simulink model "Motor_control"  (R2025b)
settings: Solver=ode45  StartTime=0.0  StopTime=3  MaxStep=1e-5  RelTol=1e-5
undefined symbols (not defined in the file): C, F, fc, G, K, K_I, L, T, x_r
settings Model: Creator=noeliarosales  LastModifiedBy=noeliarosales

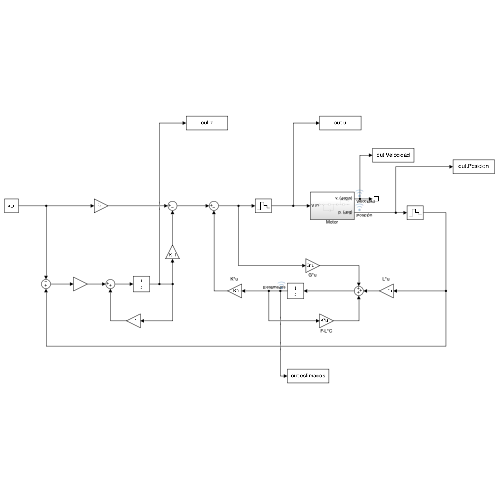
[thumbnail: Simulink's stored preview of the top-level diagram]
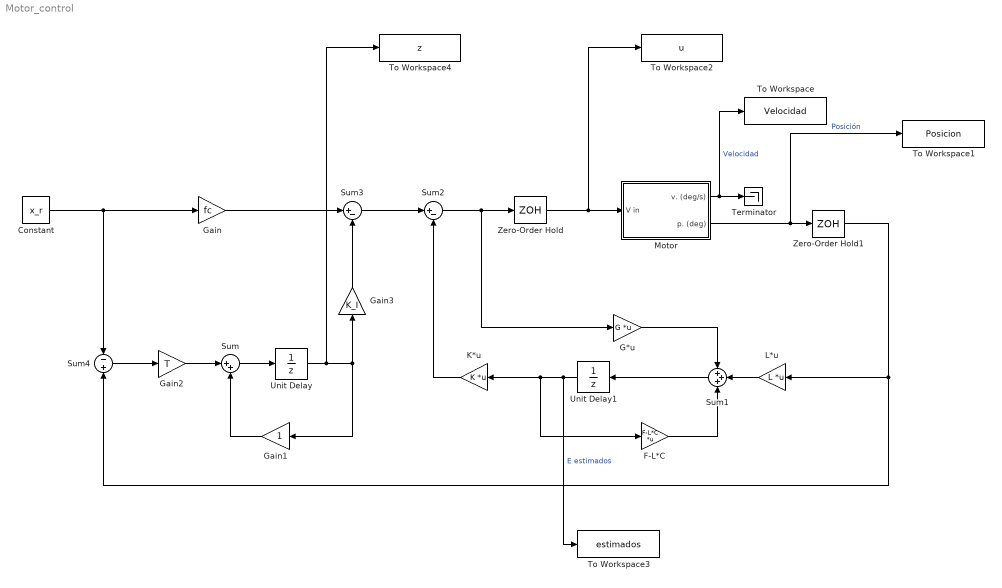
== system Motor_control ==
  Constant : Constant  Value=x_r
  F-L*C : Gain  Gain=F-L*C  Multiplication=Matrix(K*u)
  G*u : Gain  Gain=G  Multiplication=Matrix(K*u)
  Gain : Gain  Gain=fc
  Gain1 : Gain
  Gain2 : Gain  Gain=T
  Gain3 : Gain  Gain=K_I
  K*u : Gain  Gain=K  Multiplication=Matrix(K*u)
  L*u : Gain  Gain=L  Multiplication=Matrix(K*u)
  Motor : Subsystem
  Sum : Sum  Inputs=|++
  Sum1 : Sum  Inputs=+++
  Sum2 : Sum  Inputs=|+-
  Sum3 : Sum  Inputs=|+-
  Sum4 : Sum  Inputs=-+
  Terminator : Terminator
  To Workspace : ToWorkspace  VariableName=Velocidad  SaveFormat=Timeseries  SampleTime=-1
  To Workspace1 : ToWorkspace  VariableName=Posicion  SaveFormat=Timeseries  SampleTime=-1
  To Workspace2 : ToWorkspace  VariableName=u  SaveFormat=Timeseries  SampleTime=-1
  To Workspace3 : ToWorkspace  VariableName=estimados  SaveFormat=Timeseries  SampleTime=-1
  To Workspace4 : ToWorkspace  VariableName=z  SaveFormat=Timeseries  SampleTime=-1
  Unit Delay : UnitDelay  SampleTime=-1  HasFrameUpgradeWarning=on
  Unit Delay1 : UnitDelay  SampleTime=-1  HasFrameUpgradeWarning=on
  Zero-Order Hold : ZeroOrderHold  SampleTime=T
  Zero-Order Hold1 : ZeroOrderHold  SampleTime=T
  wires:
  L*u/1 -> Sum1/2
  G*u/1 -> Sum1/1
  F-L*C/1 -> Sum1/3
  Unit Delay1/1 -> To Workspace3/1, K*u/1, F-L*C/1  "E estimados"
  Sum1/1 -> Unit Delay1/1
  K*u/1 -> Sum2/2
  Sum3/1 -> Sum2/1
  Constant/1 -> Sum4/1, Gain/1
  Gain/1 -> Sum3/1
  Gain3/1 -> Sum3/2
  Unit Delay/1 -> To Workspace4/1, Gain3/1, Gain1/1
  Sum/1 -> Unit Delay/1
  Gain1/1 -> Sum/2
  Gain2/1 -> Sum/1
  Sum4/1 -> Gain2/1
  Motor/2(p. (deg)) -> To Workspace1/1, Zero-Order Hold1/1  "Posición"
  Motor/1(v. (deg/s)) -> To Workspace/1, Terminator/1  "Velocidad"
  Sum2/1 -> G*u/1, Zero-Order Hold/1
  Zero-Order Hold/1 -> To Workspace2/1, Motor/1(V in)
  Zero-Order Hold1/1 -> L*u/1, Sum4/2

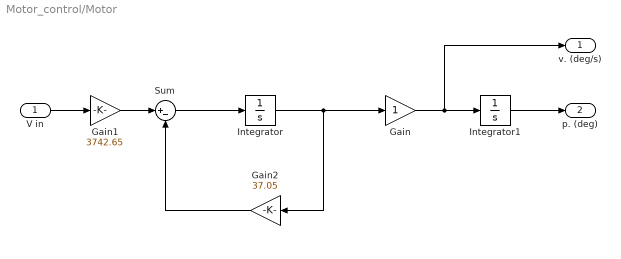
== system Motor_control/Motor ==
  V in : Inport
  Gain : Gain
  Gain1 : Gain  Gain=3742.65
  Gain2 : Gain  Gain=37.05
  Integrator : Integrator
  Integrator1 : Integrator
  Sum : Sum  Inputs=|+-
  v. (deg/s) : Outport
  p. (deg) : Outport  Port=2
  wires:
  Gain2/1 -> Sum/2
  Integrator/1 -> Gain2/1, Gain/1
  Gain1/1 -> Sum/1
  Gain/1 -> v. (deg/s)/1, Integrator1/1
  Integrator1/1 -> p. (deg)/1
  V in/1 -> Gain1/1
  Sum/1 -> Integrator/1
